simulink model "SimilinkDynamicModel"  (R2017b)
settings: Solver=VariableStepAuto  StartTime=0.0  StopTime=1000  RelTol=1e-3
settings Model: Creator=olavoie  LastModifiedBy=olavoie

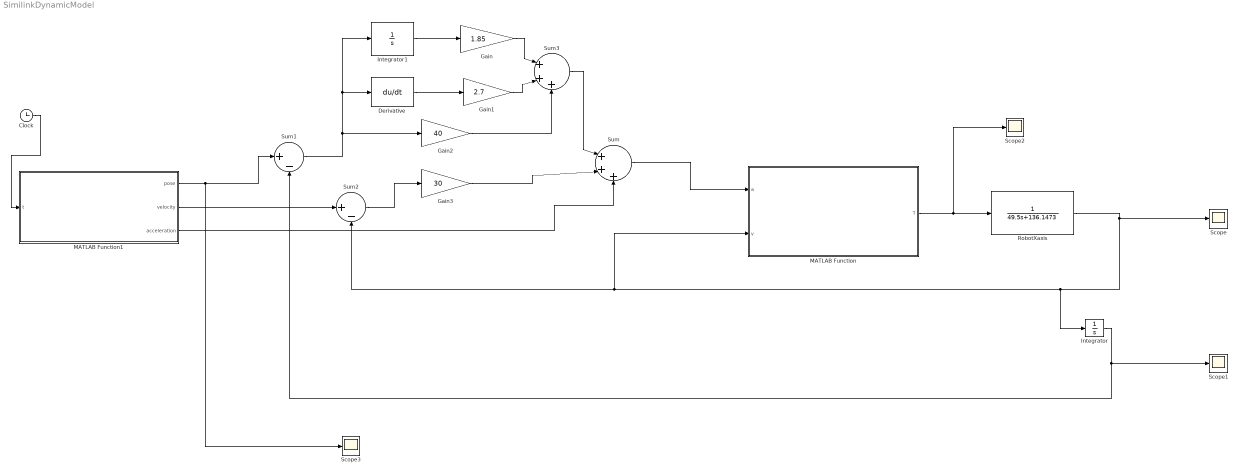
== system SimilinkDynamicModel ==
  Clock : Clock
      settings: Decimation=2
  Derivative : Derivative
  Gain : Gain  Gain=1.85
  Gain1 : Gain  Gain=2.7
  Gain2 : Gain  Gain=40
  Gain3 : Gain  Gain=30
  Integrator : Integrator
  Integrator1 : Integrator
  MATLAB Function : MATLAB Function  TreatAsAtomicUnit=on
  MATLAB Function1 : MATLAB Function  TreatAsAtomicUnit=on
  RobotXaxis : TransferFcn  Denominator=[49.5 136.1473]
  Scope{,1..3} (4 alike) : Scope
  Sum : Sum  Inputs=|+++
  Sum1 : Sum  Inputs=|+-
  Sum2 : Sum  Inputs=|+-
  Sum3 : Sum  Inputs=|+++
  wires:
  MATLAB Function1/3(acceleration) -> Sum/3
  Sum/1 -> MATLAB Function/1(a)
  Clock/1 -> MATLAB Function1/1(t)
  MATLAB Function/1(T) -> RobotXaxis/1, Scope2/1
  Sum1/1 -> Gain2/1, Derivative/1, Integrator1/1
  MATLAB Function1/1(pose) -> Scope3/1, Sum1/1
  MATLAB Function1/2(velocity) -> Sum2/1
  RobotXaxis/1 -> Integrator/1, Sum2/2, MATLAB Function/2(v), Scope/1
  Integrator/1 -> Sum1/2, Scope1/1
  Integrator1/1 -> Gain/1
  Derivative/1 -> Gain1/1
  Gain/1 -> Sum3/1
  Gain1/1 -> Sum3/2
  Sum3/1 -> Sum/1
  Gain2/1 -> Sum3/3
  Sum2/1 -> Gain3/1
  Gain3/1 -> Sum/2

== matlab function SimilinkDynamicModel/MATLAB Function1 ==
  data: pose output; velocity output; acceleration output; t input

function [pose, velocity, acceleration] = SimulinkTrajectoryGenerator(t)
    timeStamp      = 0.02;
    TrajectoryTime = 10;
    startPose      = 0;
    endPose        = 10;

    j = t * timeStamp;
    if j > TrajectoryTime
        j = TrajectoryTime;
    end
    pose         = poseTrajectory(j, startPose, endPose, TrajectoryTime);
    velocity     = velocityTrajectory(j, startPose, endPose, TrajectoryTime);
    acceleration = accelarationTrajectory(j, startPose, endPose, TrajectoryTime);
    
end


function y = poseTrajectory(t, P0, P1, timeResponse)
    spline_time_squared = t^2;
    spline_time_cubed   = t^3;
    t_f_squared = timeResponse^2;
    t_f_cubed   = timeResponse^3;
    
    y = P0 + (3 / t_f_squared) * (P1 - P0) * spline_time_squared + (-2 / t_f_cubed) * (P1 - P0) * spline_time_cubed;

end

function y = velocityTrajectory(t, P0, P1, timeResponse)
    spline_time         = t;
    spline_time_squared = t^2;
    t_f_squared = timeResponse^2;
    t_f_cubed   = timeResponse^3;
    
    y = 2 * (3 / t_f_squared) * (P1 - P0) * spline_time + 3 * (-2 / t_f_cubed) * (P1 - P0) * spline_time_squared;

end

function y = accelarationTrajectory(t, P0, P1, timeResponse)
    spline_time         = t;
    t_f_squared = timeResponse^2;
    t_f_cubed   = timeResponse^3;
    
    y = 2 * (3 / t_f_squared) * (P1 - P0) + 6 * (-2 / t_f_cubed) * (P1 - P0) * spline_time;
end

== matlab function SimilinkDynamicModel/MATLAB Function ==
  data: a input; T output; v input
function T = SimulinkDynamicModel(a, v)
    AUV_MASS               = 50.0;
    AUV_VOLUME             = 0.04949949;
    BUOYANCY_CENTER        = [0.0, 0.0, 0.0];
    X_SURFACE              = 0.73 * 0.17;
    Y_SURFACE              = X_SURFACE;
    Z_SURFACE              = X_SURFACE + Y_SURFACE;
    ROLL_SURFACE           = 0.0;
    PITCH_SURFACE          = 0.0;
    YAW_SURFACE            = 0.40 * 0.17;
    GRAVITY                = AUV_MASS * 9.81;
    BUOYANCY               = -AUV_VOLUME * 1025 * 9.81;
    resultingForce         = GRAVITY + BUOYANCY;

    ConstDragCoefficient   = [136.1473; 104.6571; 0.0; 0.0; 0.0; 76.4971];
    QuadDragCoefficient    = [3.7787; 51.7301; 0.0; 0.0; 0.0; -122.1888];
                    
    MassInertiaCoefficient = [[50, 0.0, 0.0, 0.0, 0.0, 0.0];
                             [0.0, 50, 0.0, 0.0, 0.0, 0.0];
                             [0.0, 0.0, 50, 0.0, 0.0, 0.0];
                             [0.0, 0.0, 0.0, 1.9, 0.0, 0.0];
                             [0.0, 0.0, 0.0, 0.0, 3.1, 0.0];
                             [0.0, 0.0, 0.0, 0.0, 0.0, 1.7]];
    orientation  = [0;0;0];
    velocity     = [v;0;0;0;0;0];
    acceleration = [a;0;0;0;0;0];
          
    M = MassInertiaCoefficient;    
    D = ComputeDamping(ConstDragCoefficient, QuadDragCoefficient, velocity);
    G = ComputeGravityVector(resultingForce, BUOYANCY, BUOYANCY_CENTER, orientation);

    Tt = M * acceleration + D .* velocity + G;
    T = Tt(1);
    
end

function GravityVectorT = ComputeGravityVector(resultingForce, Buoyancy, buoyancy_center, orientation)
        
        GravityVectorT = [0;0;resultingForce;0;0;0];
end

function Damping = ComputeDamping(ConstDragCoefficient, QuadDragCoefficient, Velocity)
    
    Damping = ConstDragCoefficient + QuadDragCoefficient .* (Velocity .* Velocity);
    
end
